simulink model "MidWorkSvertant"  (Simulink 8.1)
settings: Solver=ode45  StartTime=0.0  StopTime=inf  RelTol=1e-3
libraries: commdigbbndpm3 x4, commchan3 x2, commrandsrc2 x2, commcnvcod2 x2, commsink2 x2
settings Model: Creator=user  LastModifiedBy=admin
settings DataIOCC: SignalLoggingSaveFormat=Dataset
settings OptimizationCC: ExpressionDepthLimit=128
settings DebuggingCC: FcnCallInpInsideContextMsg=EnableAllAsError
settings GRTTargetCC: CombineOutputUpdateFcns=on  GRTInterface=off

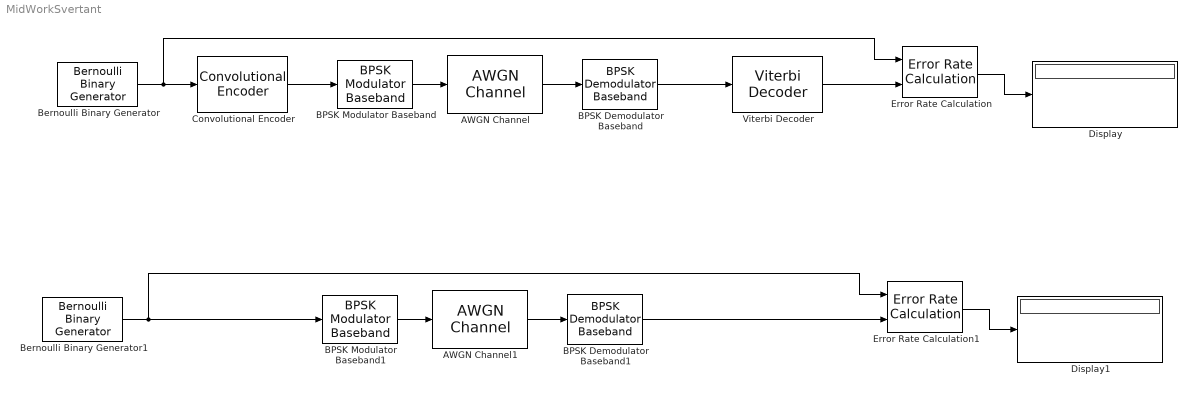
== system MidWorkSvertant ==
  AWGN Channel : commchan3/AWGN Channel  InputProcessing=Columns as channels (frame based)  seed=67  noiseMode="Signal to noise ratio  (Eb/No)"  EbNodB=2  EsNodB=10  SNRdB=10  bitsPerSym=1  Ps=1  Tsym=1  variance=1
  AWGN Channel1 : commchan3/AWGN Channel  InputProcessing=Columns as channels (frame based)  seed=67  noiseMode="Signal to noise ratio  (Eb/No)"  EbNodB=2  EsNodB=10  SNRdB=10  bitsPerSym=1  Ps=1  Tsym=1  variance=1
  BPSK Demodulator Baseband : commdigbbndpm3/BPSK Demodulator Baseband  Ph=0  DecType=Hard decision  VarSource=Dialog  Variance=1  outDtype=double  derotateFactorWordLen=16
  BPSK Demodulator Baseband1 : commdigbbndpm3/BPSK Demodulator Baseband  Ph=0  DecType=Hard decision  VarSource=Dialog  Variance=1  outDtype=double  derotateFactorWordLen=16
  BPSK Modulator Baseband : commdigbbndpm3/BPSK Modulator Baseband  Ph=0  outDtype=double  outWordLen=16  outUDDataType=sfix(16)  outFracLenMode=Best precision  outFracLen=15
  BPSK Modulator Baseband1 : commdigbbndpm3/BPSK Modulator Baseband  Ph=0  outDtype=double  outWordLen=16  outUDDataType=sfix(16)  outFracLenMode=Best precision  outFracLen=15
  Bernoulli Binary Generator : commrandsrc2/Bernoulli Binary Generator  P=0.5  seed=67  Ts=1  frameBased=off  sampPerFrame=4  orient=off  outDataType=double
  Bernoulli Binary Generator1 : commrandsrc2/Bernoulli Binary Generator  P=0.5  seed=67  Ts=1  frameBased=off  sampPerFrame=4  orient=off  outDataType=double
  Convolutional Encoder : commcnvcod2/Convolutional Encoder  trellis=poly2trellis(4, [17 15])  opMode=Continuous  DelayedResetAction=off  hasIniStPort=off  hasFinStPort=off  usePuncVector=off  punctureVector=[1; 1; 0; 1; 0; 1]  reset=Unused parameter value
  Display : Display
  Display1 : Display
  Error Rate Calculation : commsink2/Error Rate Calculation  N=20  st_delay=0  cp_mode=Entire frame  subframe=[]  PMode=Port  WsName=ErrorVec  RsMode2=off  stop=off  numErr=2  maxBits=15
  Error Rate Calculation1 : commsink2/Error Rate Calculation  N=0  st_delay=0  cp_mode=Entire frame  subframe=[]  PMode=Port  WsName=ErrorVec  RsMode2=off  stop=off  numErr=2  maxBits=15
  Viterbi Decoder : commcnvcod2/Viterbi Decoder  trellis=poly2trellis(4, [17 15])  isPunctured=off  punctureVector=[1; 1; 0; 1; 0; 1]  erasures=off  dectype=Hard decision  runSigValErrCheck=off  nsdecb=4  smWordLength=16  tbdepth=20  opmode=Continuous  reset=off  outDataType=Inherit via internal rule  delayedResetAction=off
  wires:
  Bernoulli Binary Generator/1 -> Convolutional Encoder/1, Error Rate Calculation/1
  Convolutional Encoder/1 -> BPSK Modulator Baseband/1
  BPSK Modulator Baseband/1 -> AWGN Channel/1
  AWGN Channel/1 -> BPSK Demodulator Baseband/1
  BPSK Demodulator Baseband/1 -> Viterbi Decoder/1
  Viterbi Decoder/1 -> Error Rate Calculation/2
  Error Rate Calculation/1 -> Display/1
  Bernoulli Binary Generator1/1 -> BPSK Modulator Baseband1/1, Error Rate Calculation1/1
  BPSK Modulator Baseband1/1 -> AWGN Channel1/1
  AWGN Channel1/1 -> BPSK Demodulator Baseband1/1
  BPSK Demodulator Baseband1/1 -> Error Rate Calculation1/2
  Error Rate Calculation1/1 -> Display1/1
